simulink model "RS232ex5"  (Simulink 8.7)
settings: Solver=FixedStepDiscrete  StartTime=0.0  StopTime=5  FixedStep=.5  RelTol=1e-3
libraries: RS232 x4
settings Model: Creator=Leonardo  LastModifiedBy=Leonardo
settings DataIOCC: SignalLoggingSaveFormat=ModelDataLogs  SignalLoggingName=sigsOut
settings OptimizationCC: BlockReduction=off  BooleanDataType=off
settings DebuggingCC: SaveWithParameterizedLinksMsg=none  SignalResolutionControl=TryResolveAllWithWarning  MultiTaskDSMMsg=warning  MultiTaskCondExecSysMsg=none  StrictBusMsg=None
settings HardwareCC: TargetUnknown=on
settings GRTTargetCC: GeneratePreprocessorConditionals=Use local settings  CombineOutputUpdateFcns=off  GRTInterface=on

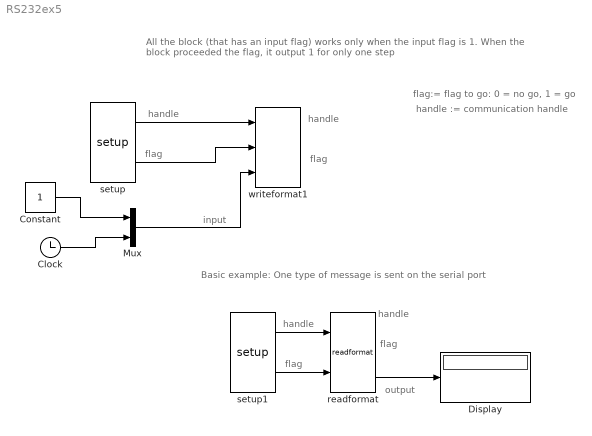
== system RS232ex5 ==
  note: All the block (that has an input flag) works only when the input flag is 1.
      | When the block proceeded the flag, it output 1 for only one step
  note: flag:= flag to go: 0 = no go, 1 = go
  note: handle := communication handle
  note: flag
  note: input
  note: handle
  note: handle
  note: flag
  note: Basic example: One type of message is sent on the serial port
  note: flag
  note: output
  note: handle
  note: flag
  note: handle
  Clock : Clock
  Constant : Constant
  Display : Display
  Mux : Mux  Inputs=2
  readformat : RS232/readformat  fmtString=00594-003+030106%03d%03d_  nCharTerm=1  sampTime=-1
  setup : RS232/setup  port=COM2  baudrate=115200  databit=8  stopbit=1  parity=None
  setup1 : RS232/setup  port=COM1  baudrate=115200  databit=8  stopbit=1  parity=None
  writeformat1 : RS232/writeformat1  fmtString=00594-003+030106%03d%03d_  sampTime=-1
  wires:
  setup/1 -> writeformat1/1
  setup/2 -> writeformat1/2
  Clock/1 -> Mux/2
  Constant/1 -> Mux/1
  Mux/1 -> writeformat1/3
  setup1/1 -> readformat/1
  setup1/2 -> readformat/2
  readformat/3 -> Display/1
